simulink model "OFDM_Tx_HW"  (R2020a)
settings: Solver=FixedStepDiscrete  StartTime=0.0  StopTime=inf  RelTol=1e-3
InitFcn:
  | % Set parameters
  | fs = 20e6;
  | fclk = 240e6;
  | ssr = 2;
  | fdc = fclk*ssr*8;
  | 
  | % Load libraries
  | addpath('./lib');
  | 
  | % Create filters
  | run ./filter_design_20mhz;
  | 
  | % Load all required variables
  | load('variables/read_addr_data');
  | load('variables/read_addr_cp');
  | load('variables/read_addr_pream');
  | load('variables/read_addr_rx');
  | load('variables/pilot');
  | load('variables/sc_index');
  | load('variables/LTSfreq');
  | load('variables/STSfreq');
  | load('variables/LTSread');
  | load('variables/STSread');
  | 
  | run ./scripts/rfgen;
values from neighbouring files (symbols this model uses):
  decimation_unique = dsp.SampleRateConverter('InputSampleRate', fdc/64,     'OutputSampleRate', fs,     'Bandwidth', fs*0.9,     'OutputRateTolerance', 0,     'StopbandAttenuation', 100)    [filter_design_20mhz.m]
  interpolation_single = dsp.SampleRateConverter('InputSampleRate', fs,     'OutputSampleRate', fclk,     'Bandwidth', fs*0.9,     'OutputRateTolerance', 0,     'StopbandAttenuation', 100)    [filter_design_20mhz.m]
  interpolation_ssr = dsp.SampleRateConverter('InputSampleRate', fclk,     'OutputSampleRate', fclk*ssr,     'Bandwidth', fs*0.9,     'OutputRateTolerance', 0,     'StopbandAttenuation', 100)    [filter_design_20mhz.m]
undefined symbols (not defined in the file or in its folder): designMultirateFIR, LTSfreq, LTSread, pilot, read_addr_cp, read_addr_data, read_addr_pream, read_addr_rx, sc_index, STSfreq, STSread
libraries: hdlsllib x87, simulink x55, xbsIndex_r4 x48, dspmlti4 x23, xrbsSSR_Library x8, dspsigops x6, dspswit3 x4, dsphdlmathfun x3, dspsigattribs x2, dsphdlxfrm x2, dsphdlsigops x1, lib_rfsignalgenerator x1
(part 2 of 6)

== system OFDM_Tx_HW/OFDMTx/DataGenerator ==
  modScheme : Inport
  dataValid : Inport  Port=2
  preambleValid : Inport  Port=3
  dataReady : Inport  Port=4
  pilotValid : Inport  Port=5
  Constant : Constant  Value=0  OutDataTypeStr=boolean  SampleTime=1/fs
  Data Multiplexer : MATLAB Function  TreatAsAtomicUnit=on
  LTSfreq : Subsystem
  PilotGen : Subsystem
  RF Signal Generator : lib_rfsignalgenerator/RF Signal Generator  SystemSampleTime=-1  Latency=0  AutoFrameSizeCalculation=off
  STSFreq : Subsystem
  dataOut : Outport  VectorParamsAs1DForOutWhenUnconnected=off
  preambValOut : Outport  Port=2  VectorParamsAs1DForOutWhenUnconnected=off
  dataValidOut : Outport  Port=3  VectorParamsAs1DForOutWhenUnconnected=off
  symValidOut : Outport  Port=4  VectorParamsAs1DForOutWhenUnconnected=off
  wires:
  dataValid/1 -> PilotGen/1(dataValidIn), dataValidOut/1
  preambleValid/1 -> STSFreq/1(preamVal), LTSfreq/1(preambVal), preambValOut/1
  LTSfreq/2(ltsVal) -> Data Multiplexer/8(ltsval)
  LTSfreq/1(ltsFreq) -> Data Multiplexer/7(lts)
  STSFreq/2(stsVal) -> Data Multiplexer/6(stsval)
  STSFreq/1(stsFreq) -> Data Multiplexer/5(sts)
  pilotValid/1 -> PilotGen/2(pilotValidIn), Data Multiplexer/4(pval)
  PilotGen/1(pilotOut) -> Data Multiplexer/3(pilots)
  RF Signal Generator/2 -> Data Multiplexer/1(symbols)
  Data Multiplexer/1(data) -> dataOut/1
  modScheme/1 -> RF Signal Generator/1
  RF Signal Generator/1 -> symValidOut/1
  Constant/1 -> RF Signal Generator/2
  dataReady/1 -> RF Signal Generator/3, Data Multiplexer/2(dataready)

== system OFDM_Tx_HW/OFDMTx/IFFT ==
  dataIn : Inport
  preambleValidIn : Inport  Port=2
  "dataValidIn " : Inport  Port=3
  Delay : Delay  DelayLength=173  InitialCondition=0  UseCircularBuffer=on
  Delay1 : Delay  DelayLength=173  InitialCondition=0  UseCircularBuffer=on
  IFFT HDL Optimized : dsphdlxfrm/IFFT HDL Optimized  FFTLength=64  Architecture=Streaming Radix 2^2  ComplexMultiplication=Use 3 multipliers and 5 adders  BitReversedOutput=off  BitReversedInput=off  Normalize=on  SimulateUsing=Code generation  RoundingMethod=Floor  ResetInputPort=off  StartOutputPort=off  EndOutputPort=off
      settings: SourceProductBaseCode=DS
  IFFTValid : Subsystem
  Terminator : Terminator
  dataOut : Outport  VectorParamsAs1DForOutWhenUnconnected=off
  preambValidOut : Outport  Port=2  VectorParamsAs1DForOutWhenUnconnected=off
  dataValidOut : Outport  Port=3  VectorParamsAs1DForOutWhenUnconnected=off
  wires:
  dataIn/1 -> IFFT HDL Optimized/1
  IFFT HDL Optimized/2 -> Terminator/1
  "dataValidIn "/1 -> IFFTValid/2(dataValid), Delay1/1
  IFFTValid/1(ifftValid) -> IFFT HDL Optimized/2
  preambleValidIn/1 -> IFFTValid/1(preambleValid), Delay/1
  Delay/1 -> preambValidOut/1
  Delay1/1 -> dataValidOut/1
  IFFT HDL Optimized/1 -> dataOut/1

== system OFDM_Tx_HW/OFDMTx/SCMapper ==
  dataIn : Inport
  preambValid : Inport  Port=2
  dataValid : Inport  Port=3
  DataMapper : Subsystem
  Mux2 : MATLAB Function  TreatAsAtomicUnit=on
  PremableMapper : Subsystem
  dataOut : Outport  VectorParamsAs1DForOutWhenUnconnected=off
  preambValidOut : Outport  Port=2  VectorParamsAs1DForOutWhenUnconnected=off
  dataValidOut : Outport  Port=3  VectorParamsAs1DForOutWhenUnconnected=off
  wires:
  PremableMapper/1(preambleShiftOut) -> Mux2/1(preamb)
  PremableMapper/2(preambValOut) -> preambValidOut/1, Mux2/2(preambVal)
  DataMapper/1(dataOut) -> Mux2/3(data)
  DataMapper/2(dataValidOut) -> dataValidOut/1, Mux2/4(dataVal)
  dataIn/1 -> DataMapper/1(dataIn), PremableMapper/1(data)
  preambValid/1 -> PremableMapper/2(preambVal)
  dataValid/1 -> DataMapper/2(dataValid)
  Mux2/1(dataOut) -> dataOut/1

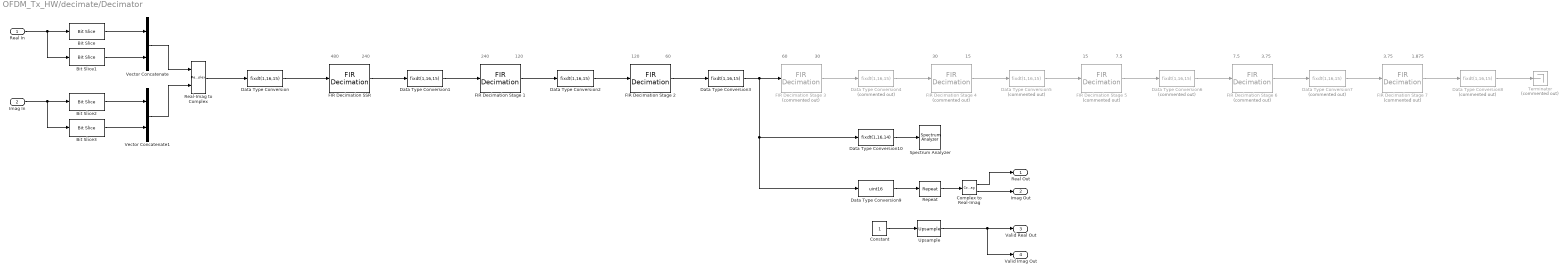
== system OFDM_Tx_HW/decimate/Decimator ==
  note: 1.875
  note: 3.75
  note: 3.75
  note: 7.5
  note: 7.5
  note: 15
  note: 15
  note: 30
  note: 30
  note: 480
  note: 240
  note: 240
  note: 120
  note: 120
  note: 60
  note: 60
  Real In : Inport
  Imag In : Inport  Port=2
  Bit Slice : hdlsllib/Logic and Bit Operations/Bit Slice  lidx=15  ridx=0
      settings: SourceProductBaseCode=SL
  Bit Slice1 : hdlsllib/Logic and Bit Operations/Bit Slice  lidx=31  ridx=16
      settings: SourceProductBaseCode=SL
  Bit Slice2 : hdlsllib/Logic and Bit Operations/Bit Slice  lidx=15  ridx=0
      settings: SourceProductBaseCode=SL
  Bit Slice3 : hdlsllib/Logic and Bit Operations/Bit Slice  lidx=31  ridx=16
      settings: SourceProductBaseCode=SL
  Complex to Real-Imag : ComplexToRealImag
  Constant : Constant  OutDataTypeStr=boolean  SampleTime=1/(fclk/4)
  Data Type Conversion : DataTypeConversion  OutDataTypeStr=fixdt(1,16,15)  ConvertRealWorld=Stored Integer (SI)
  Data Type Conversion1 : DataTypeConversion  OutDataTypeStr=fixdt(1,16,15)  RndMeth=Round  SaturateOnIntegerOverflow=on
  Data Type Conversion10 : DataTypeConversion  OutDataTypeStr=fixdt(1,16,14)  ConvertRealWorld=Stored Integer (SI)
  Data Type Conversion2 : DataTypeConversion  OutDataTypeStr=fixdt(1,16,15)  RndMeth=Round  SaturateOnIntegerOverflow=on
  Data Type Conversion3 : DataTypeConversion  OutDataTypeStr=fixdt(1,16,15)  RndMeth=Round  SaturateOnIntegerOverflow=on
  Data Type Conversion{4..8} (5 alike) : DataTypeConversion  Commented=on  OutDataTypeStr=fixdt(1,16,15)  RndMeth=Round  SaturateOnIntegerOverflow=on
  Data Type Conversion9 : DataTypeConversion  OutDataTypeStr=uint16  ConvertRealWorld=Stored Integer (SI)
  FIR Decimation SSR : dspmlti4/FIR Decimation  FilterSource=Dialog parameters  h=decimation_ssr.Numerator  D=2  filtStruct=Direct form  FilterObject=FDECIM  InputProcessing=Columns as channels (frame based)  framing=Enforce single-rate processing  inputOffset=0  outputBufInitCond=0  roundingMode=Floor  overflowMode=off  firstCoeffDataTypeStr=Inherit: Same word length as input  firstCoeffMin=[]  firstCoeffMax=[]  firstCoeffLastDataTypeStr=Inherit: Same word length as input  outputDataTypeStr=Inherit: Same as product output  outputMin=[]  outputMax=[]  outputLastDataTypeStr=Inherit: Same as product output
  FIR Decimation Stage 1 : dspmlti4/FIR Decimation  FilterSource=Dialog parameters  h=decimation_single.Numerator  D=2  filtStruct=Direct form  FilterObject=FDECIM  framing=Enforce single-rate processing  inputOffset=0  outputBufInitCond=0  roundingMode=Floor  overflowMode=off  firstCoeffDataTypeStr=Inherit: Same word length as input  firstCoeffMin=[]  firstCoeffMax=[]  firstCoeffLastDataTypeStr=Inherit: Same word length as input  outputDataTypeStr=Inherit: Same as product output  outputMin=[]  outputMax=[]  outputLastDataTypeStr=Inherit: Same as product output
  FIR Decimation Stage 2 : dspmlti4/FIR Decimation  FilterSource=Dialog parameters  h=decimation_single.Numerator  D=2  filtStruct=Direct form  FilterObject=FDECIM  framing=Enforce single-rate processing  inputOffset=0  outputBufInitCond=0  roundingMode=Floor  overflowMode=off  firstCoeffDataTypeStr=Inherit: Same word length as input  firstCoeffMin=[]  firstCoeffMax=[]  firstCoeffLastDataTypeStr=Inherit: Same word length as input  outputDataTypeStr=Inherit: Same as product output  outputMin=[]  outputMax=[]  outputLastDataTypeStr=Inherit: Same as product output
  FIR Decimation Stage {3..7} (5 alike) : dspmlti4/FIR Decimation  Commented=on  FilterSource=Dialog parameters  h=decimation_single.Numerator  D=2  filtStruct=Direct form  FilterObject=FDECIM  framing=Enforce single-rate processing  inputOffset=0  outputBufInitCond=0  roundingMode=Floor  overflowMode=off  firstCoeffDataTypeStr=Inherit: Same word length as input  firstCoeffMin=[]  firstCoeffMax=[]  firstCoeffLastDataTypeStr=Inherit: Same word length as input  outputDataTypeStr=Inherit: Same as product output  outputMin=[]  outputMax=[]  outputLastDataTypeStr=Inherit: Same as product output
  Real-Imag to Complex : RealImagToComplex
  Repeat : dspsigops/Repeat  N=4  RateOptions=Allow multirate processing  ic=0  mode=Unused parameter value
  Spectrum Analyzer : SpectrumAnalyzer
  Terminator : Terminator  Commented=on
  Upsample : dspsigops/Upsample  N=4  phase=0  RateOptions=Allow multirate processing  ic=0  mode=Unused parameter value
  Vector Concatenate : Concatenate
  Vector Concatenate1 : Concatenate
  Real Out : Outport
  Imag Out : Outport  Port=2
  Valid Real Out : Outport  Port=3
  Valid Imag Out : Outport  Port=4
  wires:
  Data Type Conversion8/1 -> Terminator/1
  Data Type Conversion3/1 -> Data Type Conversion10/1, Data Type Conversion9/1, FIR Decimation Stage 3/1
  Data Type Conversion10/1 -> Spectrum Analyzer/1
  Upsample/1 -> Valid Real Out/1, Valid Imag Out/1
  Data Type Conversion9/1 -> Repeat/1
  Repeat/1 -> Complex to Real-Imag/1
  Data Type Conversion2/1 -> FIR Decimation Stage 2/1
  FIR Decimation Stage 6/1 -> Data Type Conversion7/1
  Data Type Conversion1/1 -> FIR Decimation Stage 1/1
  FIR Decimation Stage 1/1 -> Data Type Conversion2/1
  Complex to Real-Imag/2 -> Imag Out/1
  Vector Concatenate1/1 -> Real-Imag to Complex/2
  Vector Concatenate/1 -> Real-Imag to Complex/1
  Real-Imag to Complex/1 -> Data Type Conversion/1
  Bit Slice1/1 -> Vector Concatenate/2
  FIR Decimation Stage 5/1 -> Data Type Conversion6/1
  Bit Slice/1 -> Vector Concatenate/1
  FIR Decimation SSR/1 -> Data Type Conversion1/1
  FIR Decimation Stage 7/1 -> Data Type Conversion8/1
  Real In/1 -> Bit Slice/1, Bit Slice1/1
  Data Type Conversion6/1 -> FIR Decimation Stage 6/1
  FIR Decimation Stage 2/1 -> Data Type Conversion3/1
  Data Type Conversion7/1 -> FIR Decimation Stage 7/1
  Bit Slice2/1 -> Vector Concatenate1/1
  Constant/1 -> Upsample/1
  Imag In/1 -> Bit Slice3/1, Bit Slice2/1
  FIR Decimation Stage 4/1 -> Data Type Conversion5/1
  Data Type Conversion/1 -> FIR Decimation SSR/1
  Bit Slice3/1 -> Vector Concatenate1/2
  FIR Decimation Stage 3/1 -> Data Type Conversion4/1
  Complex to Real-Imag/1 -> Real Out/1
  Data Type Conversion5/1 -> FIR Decimation Stage 5/1
  Data Type Conversion4/1 -> FIR Decimation Stage 4/1

== system OFDM_Tx_HW/decimate/Unique Decimation ==
  Real In : Inport
  Imag In : Inport  Port=2
  Valid Real In : Inport  Port=3
  Valid Imag In : Inport  Port=4
  Unique Decimation : Subsystem  VariantControl=SystemGenerator
  Unique Decimation1 : Subsystem  VariantControl=Simulink
  Data : Outport
  Valid : Outport  Port=2

== system OFDM_Tx_HW/interpolate/interpolate ==
  s_tdata : Inport
  s_tvalid : Inport  Port=2
  Convert To AXI-Stream : Subsystem
  Data Type Conversion2 : DataTypeConversion  OutDataTypeStr=uint64
  Data Type Conversion8 : DataTypeConversion  OutDataTypeStr=boolean
  FIR Interpolation SSR : Subsystem
  FIR Interpolation Single : Subsystem
  Imag Slice : xbsIndex_r4/Slice  nbits=1  boolean_output=off  mode=Two Bit Locations  bit1=31  base1=LSB of Input  bit0=16  base0=LSB of Input  dbl_ovrd=off  block_type=slice
  Real Slice : xbsIndex_r4/Slice  nbits=1  boolean_output=off  mode=Two Bit Locations  bit1=15  base1=LSB of Input  bit0=0  base0=LSB of Input  dbl_ovrd=off  block_type=slice
  Reinterpret : xbsIndex_r4/Reinterpret  force_arith_type=on  arith_type="Signed  (2's comp)"  force_bin_pt=on  bin_pt=14  block_type=reinterpret
  Reinterpret1 : xbsIndex_r4/Reinterpret  force_arith_type=on  arith_type="Signed  (2's comp)"  force_bin_pt=on  bin_pt=14  block_type=reinterpret
  Terminator : Terminator
  data : xbsIndex_r4/Gateway In  gui_display_data_type=Fixed-point  arith_type=Unsigned  n_bits=32  bin_pt=0  preci_type=Single  exp_width=8  frac_width=24  rows=1  columns=1  quantization="Round  (unbiased: +/- Inf)"  overflow=Saturate  period=1/(fs)  UseAsADC=off  ADCChannel='1'  interface=None  automatic_assignment=on  address_offset=hex2dec('00')  intf_name=''  intf_description=''  default_value=0  timing_constraint=None  locs_specified=off  LOCs={}  io_standard={}  inherit_from_input=off  hdl_port=on  dbl_ovrd=off  block_type=gatewayin
  m_axis_tdata : xbsIndex_r4/Gateway Out  inherit_from_input=on  hdl_port=on  rows=1  columns=1  UseAsDAC=off  DACChannel='1'  interface=None  automatic_assignment=on  address_offset=hex2dec('00')  intf_name=''  intf_description=''  timing_constraint=None  locs_specified=off  LOCs={}  io_standard={}  block_type=gatewayout
  m_axis_tvalid : xbsIndex_r4/Gateway Out  inherit_from_input=off  hdl_port=on  rows=1  columns=1  UseAsDAC=off  DACChannel='1'  interface=None  automatic_assignment=on  address_offset=hex2dec('00')  intf_name=''  intf_description=''  timing_constraint=None  locs_specified=off  LOCs={}  io_standard={}  block_type=gatewayout
  valid : xbsIndex_r4/Gateway In  gui_display_data_type=Boolean  arith_type=Boolean  n_bits=32  bin_pt=0  preci_type=Single  exp_width=8  frac_width=24  rows=1  columns=1  quantization="Round  (unbiased: +/- Inf)"  overflow=Saturate  period=1/(fs)  UseAsADC=off  ADCChannel='1'  interface=None  automatic_assignment=on  address_offset=hex2dec('00')  intf_name=''  intf_description=''  default_value=0  timing_constraint=None  locs_specified=off  LOCs={}  io_standard={}  inherit_from_input=off  hdl_port=on  dbl_ovrd=off  block_type=gatewayin
  m_tdata : Outport
  m_tvalid : Outport  Port=2
  wires:
  Data Type Conversion8/1 -> m_tvalid/1
  s_tvalid/1 -> valid/1
  Data Type Conversion2/1 -> m_tdata/1
  m_axis_tdata/1 -> Data Type Conversion2/1
  m_axis_tvalid/1 -> Data Type Conversion8/1
  s_tdata/1 -> data/1
  valid/1 -> Terminator/1
  data/1 -> Imag Slice/1, Real Slice/1
  Real Slice/1 -> Reinterpret/1
  Imag Slice/1 -> Reinterpret1/1
  Reinterpret/1 -> FIR Interpolation Single/1(Real In)
  Reinterpret1/1 -> FIR Interpolation Single/2(Imag In)
  FIR Interpolation Single/1(Real Out) -> FIR Interpolation SSR/1(Real In)
  FIR Interpolation Single/2(Imag Out) -> FIR Interpolation SSR/2(Imag In)
  FIR Interpolation SSR/1(Real Out) -> Convert To AXI-Stream/1(Real In)
  FIR Interpolation SSR/2(Imag Out) -> Convert To AXI-Stream/2(Imag In)
  Convert To AXI-Stream/1(Data Out) -> m_axis_tdata/1
  Convert To AXI-Stream/2(Valid Out) -> m_axis_tvalid/1

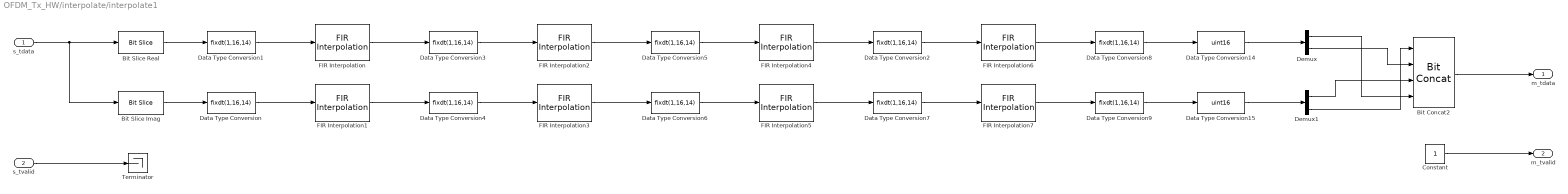
== system OFDM_Tx_HW/interpolate/interpolate1 ==
  s_tdata : Inport
  s_tvalid : Inport  Port=2
  Bit Concat2 : hdlsllib/Logic and Bit Operations/Bit Concat  numInputs=4
  Bit Slice Imag : hdlsllib/Logic and Bit Operations/Bit Slice  lidx=31  ridx=16
      settings: SourceProductBaseCode=SL
  Bit Slice Real : hdlsllib/Logic and Bit Operations/Bit Slice  lidx=15  ridx=0
      settings: SourceProductBaseCode=SL
  Constant : Constant  OutDataTypeStr=boolean  SampleTime=1/fclk
  Data Type Conversion : DataTypeConversion  OutDataTypeStr=fixdt(1,16,14)  ConvertRealWorld=Stored Integer (SI)
  Data Type Conversion1 : DataTypeConversion  OutDataTypeStr=fixdt(1,16,14)  ConvertRealWorld=Stored Integer (SI)
  Data Type Conversion14 : DataTypeConversion  OutDataTypeStr=uint16  ConvertRealWorld=Stored Integer (SI)
  Data Type Conversion15 : DataTypeConversion  OutDataTypeStr=uint16  ConvertRealWorld=Stored Integer (SI)
  Data Type Conversion{2..9} (8 alike) : DataTypeConversion  OutDataTypeStr=fixdt(1,16,14)  RndMeth=Round  SaturateOnIntegerOverflow=on
  Demux : Demux  Outputs=2
  Demux1 : Demux  Outputs=2
  FIR Interpolation : dspmlti4/FIR Interpolation  FilterSource=Dialog parameters  PrivateCoeffs=0  h=interpolation_single.getFilters.Stage1.Numerator  L=interpolation_single.getFilters.Stage1.InterpolationFactor  FilterObject=FINTERP  framing=Allow multirate processing  outputBufInitCond=0  roundingMode=Floor  overflowMode=off  firstCoeffDataTypeStr=Inherit: Same word length as input  firstCoeffMin=[]  firstCoeffMax=[]  firstCoeffLastDataTypeStr=Inherit: Same word length as input  outputDataTypeStr=Inherit: Same as product output  outputMin=[]  outputMax=[]  outputLastDataTypeStr=Inherit: Same as product output
  FIR Interpolation1 : dspmlti4/FIR Interpolation  FilterSource=Dialog parameters  PrivateCoeffs=0  h=interpolation_single.getFilters.Stage1.Numerator  L=interpolation_single.getFilters.Stage1.InterpolationFactor  FilterObject=FINTERP  framing=Allow multirate processing  outputBufInitCond=0  roundingMode=Floor  overflowMode=off  firstCoeffDataTypeStr=Inherit: Same word length as input  firstCoeffMin=[]  firstCoeffMax=[]  firstCoeffLastDataTypeStr=Inherit: Same word length as input  outputDataTypeStr=Inherit: Same as product output  outputMin=[]  outputMax=[]  outputLastDataTypeStr=Inherit: Same as product output
  FIR Interpolation2 : dspmlti4/FIR Interpolation  FilterSource=Dialog parameters  PrivateCoeffs=0  h=interpolation_single.getFilters.Stage2.Numerator  L=interpolation_single.getFilters.Stage2.InterpolationFactor  FilterObject=FINTERP  framing=Enforce single-rate processing  outputBufInitCond=0  roundingMode=Floor  overflowMode=off  firstCoeffDataTypeStr=Inherit: Same word length as input  firstCoeffMin=[]  firstCoeffMax=[]  firstCoeffLastDataTypeStr=Inherit: Same word length as input  outputDataTypeStr=Inherit: Same as product output  outputMin=[]  outputMax=[]  outputLastDataTypeStr=Inherit: Same as product output
  FIR Interpolation3 : dspmlti4/FIR Interpolation  FilterSource=Dialog parameters  PrivateCoeffs=0  h=interpolation_single.getFilters.Stage2.Numerator  L=interpolation_single.getFilters.Stage2.InterpolationFactor  FilterObject=FINTERP  framing=Enforce single-rate processing  outputBufInitCond=0  roundingMode=Floor  overflowMode=off  firstCoeffDataTypeStr=Inherit: Same word length as input  firstCoeffMin=[]  firstCoeffMax=[]  firstCoeffLastDataTypeStr=Inherit: Same word length as input  outputDataTypeStr=Inherit: Same as product output  outputMin=[]  outputMax=[]  outputLastDataTypeStr=Inherit: Same as product output
  FIR Interpolation4 : dspmlti4/FIR Interpolation  FilterSource=Dialog parameters  PrivateCoeffs=0  h=interpolation_single.getFilters.Stage3.Numerator  L=interpolation_single.getFilters.Stage3.InterpolationFactor  FilterObject=FINTERP  framing=Enforce single-rate processing  outputBufInitCond=0  roundingMode=Floor  overflowMode=off  firstCoeffDataTypeStr=Inherit: Same word length as input  firstCoeffMin=[]  firstCoeffMax=[]  firstCoeffLastDataTypeStr=Inherit: Same word length as input  outputDataTypeStr=Inherit: Same as product output  outputMin=[]  outputMax=[]  outputLastDataTypeStr=Inherit: Same as product output
  FIR Interpolation5 : dspmlti4/FIR Interpolation  FilterSource=Dialog parameters  PrivateCoeffs=0  h=interpolation_single.getFilters.Stage3.Numerator  L=interpolation_single.getFilters.Stage3.InterpolationFactor  FilterObject=FINTERP  framing=Enforce single-rate processing  outputBufInitCond=0  roundingMode=Floor  overflowMode=off  firstCoeffDataTypeStr=Inherit: Same word length as input  firstCoeffMin=[]  firstCoeffMax=[]  firstCoeffLastDataTypeStr=Inherit: Same word length as input  outputDataTypeStr=Inherit: Same as product output  outputMin=[]  outputMax=[]  outputLastDataTypeStr=Inherit: Same as product output
  FIR Interpolation6 : dspmlti4/FIR Interpolation  FilterSource=Dialog parameters  PrivateCoeffs=0  h=interpolation_ssr.getFilters.Stage1.Numerator  L=interpolation_ssr.getFilters.Stage1.InterpolationFactor  FilterObject=FINTERP  InputProcessing=Columns as channels (frame based)  framing=Enforce single-rate processing  outputBufInitCond=0  roundingMode=Floor  overflowMode=off  firstCoeffDataTypeStr=Inherit: Same word length as input  firstCoeffMin=[]  firstCoeffMax=[]  firstCoeffLastDataTypeStr=Inherit: Same word length as input  outputDataTypeStr=Inherit: Same as product output  outputMin=[]  outputMax=[]  outputLastDataTypeStr=Inherit: Same as product output
  FIR Interpolation7 : dspmlti4/FIR Interpolation  FilterSource=Dialog parameters  PrivateCoeffs=0  h=interpolation_ssr.getFilters.Stage1.Numerator  L=interpolation_ssr.getFilters.Stage1.InterpolationFactor  FilterObject=FINTERP  InputProcessing=Columns as channels (frame based)  framing=Enforce single-rate processing  outputBufInitCond=0  roundingMode=Floor  overflowMode=off  firstCoeffDataTypeStr=Inherit: Same word length as input  firstCoeffMin=[]  firstCoeffMax=[]  firstCoeffLastDataTypeStr=Inherit: Same word length as input  outputDataTypeStr=Inherit: Same as product output  outputMin=[]  outputMax=[]  outputLastDataTypeStr=Inherit: Same as product output
  Terminator : Terminator
  m_tdata : Outport
  m_tvalid : Outport  Port=2
  wires:
  Data Type Conversion9/1 -> Data Type Conversion15/1
  Data Type Conversion8/1 -> Data Type Conversion14/1
  Data Type Conversion2/1 -> FIR Interpolation6/1
  Data Type Conversion7/1 -> FIR Interpolation7/1
  FIR Interpolation7/1 -> Data Type Conversion9/1
  FIR Interpolation6/1 -> Data Type Conversion8/1
  Data Type Conversion6/1 -> FIR Interpolation5/1
  Data Type Conversion5/1 -> FIR Interpolation4/1
  FIR Interpolation4/1 -> Data Type Conversion2/1
  FIR Interpolation5/1 -> Data Type Conversion7/1
  Demux1/2 -> Bit Concat2/1
  FIR Interpolation/1 -> Data Type Conversion3/1
  Demux/2 -> Bit Concat2/2
  Demux/1 -> Bit Concat2/4
  Data Type Conversion14/1 -> Demux/1
  Data Type Conversion15/1 -> Demux1/1
  FIR Interpolation3/1 -> Data Type Conversion6/1
  Data Type Conversion3/1 -> FIR Interpolation2/1
  FIR Interpolation1/1 -> Data Type Conversion4/1
  Bit Slice Imag/1 -> Data Type Conversion/1
  Data Type Conversion1/1 -> FIR Interpolation/1
  FIR Interpolation2/1 -> Data Type Conversion5/1
  Bit Slice Real/1 -> Data Type Conversion1/1
  s_tdata/1 -> Bit Slice Imag/1, Bit Slice Real/1
  Data Type Conversion4/1 -> FIR Interpolation3/1
  s_tvalid/1 -> Terminator/1
  Data Type Conversion/1 -> FIR Interpolation1/1
  Demux1/1 -> Bit Concat2/3
  Bit Concat2/1 -> m_tdata/1
  Constant/1 -> m_tvalid/1

== system OFDM_Tx_HW/Channel/RF-ADC/Decimation Filter ==
  Data In : Inport
  FIR 0 : dspmlti4/FIR Decimation  FilterSource=Filter object  h=designMultirateFIR(1,2)  D=2  filtStruct=Direct form  FilterObject=fir0  InputProcessing=Columns as channels (frame based)  framing=Allow multirate processing  inputOffset=0  outputBufInitCond=0  roundingMode=Floor  overflowMode=off  firstCoeffDataTypeStr=Inherit: Same word length as input  firstCoeffMin=[]  firstCoeffMax=[]  firstCoeffLastDataTypeStr=Inherit: Same word length as input  outputDataTypeStr=Inherit: Same as accumulator  outputMin=[]  outputMax=[]  outputLastDataTypeStr=Inherit: Same as accumulator
  FIR 1 : dspmlti4/FIR Decimation  Commented=through  FilterSource=Filter object  h=designMultirateFIR(1,2)  D=2  filtStruct=Direct form  FilterObject=fir1  InputProcessing=Columns as channels (frame based)  framing=Allow multirate processing  inputOffset=0  outputBufInitCond=0  roundingMode=Floor  overflowMode=off  firstCoeffDataTypeStr=Inherit: Same word length as input  firstCoeffMin=[]  firstCoeffMax=[]  firstCoeffLastDataTypeStr=Inherit: Same word length as input  outputDataTypeStr=Inherit: Same as accumulator  outputMin=[]  outputMax=[]  outputLastDataTypeStr=Inherit: Same as accumulator
  FIR 2 : dspmlti4/FIR Decimation  Commented=through  FilterSource=Filter object  h=designMultirateFIR(1,2)  D=2  filtStruct=Direct form  FilterObject=fir2  InputProcessing=Columns as channels (frame based)  framing=Allow multirate processing  inputOffset=0  outputBufInitCond=0  roundingMode=Floor  overflowMode=off  firstCoeffDataTypeStr=Inherit: Same word length as input  firstCoeffMin=[]  firstCoeffMax=[]  firstCoeffLastDataTypeStr=Inherit: Same word length as input  outputDataTypeStr=Inherit: Same as accumulator  outputMin=[]  outputMax=[]  outputLastDataTypeStr=Inherit: Same as accumulator
  Data Out : Outport  VectorParamsAs1DForOutWhenUnconnected=off
  wires:
  FIR 2/1 -> Data Out/1
  Data In/1 -> FIR 0/1
  FIR 0/1 -> FIR 1/1
  FIR 1/1 -> FIR 2/1

== system OFDM_Tx_HW/Channel/RF-ADC/NCO and Mixer ==
  Data In : Inport
  Constant1 : Constant  Value=m  OutDataTypeStr=fixdt(0,2,0)  SampleTime=-1
  Data Type Conversion : DataTypeConversion  OutDataTypeStr=fixdt(1,16,15)
  Multiport Switch1 : MultiPortSwitch  DataPortOrder=Zero-based contiguous  zeroidx=on
  RF-ADC Coarse Mixer : Subsystem
  RF-ADC Fine Mixer : Subsystem
  Real-Imag to Complex : RealImagToComplex
  Data Out : Outport  VectorParamsAs1DForOutWhenUnconnected=off
  wires:
  Multiport Switch1/1 -> Data Out/1
  RF-ADC Fine Mixer/1(Data Out) -> Multiport Switch1/4
  Real-Imag to Complex/1 -> Data Type Conversion/1
  RF-ADC Coarse Mixer/1(Data Out) -> Multiport Switch1/3
  Data In/1 -> Real-Imag to Complex/1, RF-ADC Coarse Mixer/1(Data In), RF-ADC Fine Mixer/1(Data In), Real-Imag to Complex/2
  Constant1/1 -> Multiport Switch1/1
  Data Type Conversion/1 -> Multiport Switch1/2

== system OFDM_Tx_HW/Channel/RF-ADC/RF-ADC ==
  Data In : Inport
  Buffer : Buffer  N=ssr  OutputFrames=off
  Data Type Conversion : DataTypeConversion  OutDataTypeStr=fixdt(1,12,11)  SaturateOnIntegerOverflow=on
  Rate Transition : RateTransition  OutPortSampleTime=1/fs
  Data Out : Outport  VectorParamsAs1DForOutWhenUnconnected=off
  wires:
  Rate Transition/1 -> Data Type Conversion/1
  Data In/1 -> Rate Transition/1
  Data Type Conversion/1 -> Buffer/1
  Buffer/1 -> Data Out/1

== system OFDM_Tx_HW/Channel/RF-ADC/SSR Converter RF-ADC ==
  Real In : Inport
  Imag In : Inport  Port=2
  Constant : Constant  OutDataTypeStr=boolean  SampleTime=-1
  Convert 2-D to 1-D : dspsigattribs/Convert 2-D to 1-D
      settings: SourceProductBaseCode=DS
  Convert 2-D to 1-D1 : dspsigattribs/Convert 2-D to 1-D
      settings: SourceProductBaseCode=DS
  Vector to SSR Imag : Subsystem  mask{N=8, hN=8}
      mask prompts: N "Samples per clock cycle:"
      mask init:
      | if ~isequal(get_param(gcb, 'N'), get_param(gcb, 'hN'))
      |     % Delete all blocks except input and output ports
      |     delete_block(setxor(setdiff(...
      |         find_system(gcb,'LookUnderMasks','on'),...
      |         {[gcb, '/Vector'], [gcb, '/SSR']}), gcb));
      | 
      |     % Delete all wires
      |     delete_line(find_system(gcb, 'FindAll', 'on', 'LookUnderMasks',...
      |         'on', 'SearchDepth', 3, 'Type', 'line', 'Connected', 'off'));
      | 
      |     % Add the bit concatenation block
      |     add_block('hdlsllib/Logic and Bit Operations/Bit Concat',...
      |         [gcb, '/Bit Concat'],...
      |         'Position', [155 55 205 330]);
      |     set_param([gcb, '/Bit Concat'], 'numInputs', num2str(N));
      | 
      |     % Add wire to output
      |     add_line(gcb, 'Bit Concat/1', 'SSR/1');
      | 
      |     % Add selector blocks and connect wires
      |     for i = 0:N-1
      |         add_block('simulink/Signal Routing/Selector',...
      |             [gcb, '/Selector', num2str(i)],...
      |             'Position', [0 82+i*90 45 128+i*90]);
      |         set_param([gcb, '/Selector', num2str(i)], 'InputPortWidth', num2str(N), 'IndexParamArray', {num2str(N-i)});
      |         add_line(gcb, 'Vector/1', ['Selector', num2str(i), '/1'],...
      |             'autorouting', 'on');
      |         add_line(gcb, ['Selector', num2str(i), '/1'],...
      |             ['Bit Concat/', num2str(i+1)],...
      |             'autorouting', 'on');
      |     end
      |     
      |     % Set the hidden attribute to prevent unnecessary changes in
      |     % architecture while generating HDL Code.
      |     set_param(gcb, 'hN', get_param(gcb, 'N'));
      | end
      mask DialogControl DescGroupVar Prompt: Vector to SSR
      mask DialogControl DescTextVar Prompt: Convert a vector of inputs into SSR format.
  Vector to SSR Real : Subsystem  mask{N=8, hN=8}
      mask prompts: N "Samples per clock cycle:"
      mask init: same as OFDM_Tx_HW/Channel/RF-ADC/SSR Converter RF-ADC/Vector to SSR Imag
      mask DialogControl DescGroupVar Prompt: Vector to SSR
      mask DialogControl DescTextVar Prompt: Convert a vector of inputs into SSR format.
  Valid Real : Outport
  Valid Imag : Outport  Port=2
  Real Out : Outport  Port=3
  Imag Out : Outport  Port=4
  wires:
  Real In/1 -> Convert 2-D to 1-D/1
  Imag In/1 -> Convert 2-D to 1-D1/1
  Convert 2-D to 1-D/1 -> Vector to SSR Real/1(Vector)
  Convert 2-D to 1-D1/1 -> Vector to SSR Imag/1(Vector)
  Vector to SSR Real/1(SSR) -> Real Out/1
  Vector to SSR Imag/1(SSR) -> Imag Out/1
  Constant/1 -> Valid Imag/1, Valid Real/1

== system OFDM_Tx_HW/Channel/RF-DAC/Interpolation Filter ==
  Data In : Inport
  FIR 0 : dspmlti4/FIR Interpolation  Commented=through  FilterSource=Filter object  PrivateCoeffs=0  h=designMultirateFIR(3,1)  L=2  FilterObject=fir0  InputProcessing=Columns as channels (frame based)  framing=Allow multirate processing  outputBufInitCond=0  roundingMode=Floor  overflowMode=off  firstCoeffDataTypeStr=Inherit: Same word length as input  firstCoeffMin=[]  firstCoeffMax=[]  firstCoeffLastDataTypeStr=Inherit: Same word length as input  outputDataTypeStr=Inherit: Same as accumulator  outputMin=[]  outputMax=[]  outputLastDataTypeStr=Inherit: Same as accumulator
  FIR 1 : dspmlti4/FIR Interpolation  FilterSource=Filter object  PrivateCoeffs=0  h=designMultirateFIR(3,1)  L=2  FilterObject=fir1  InputProcessing=Columns as channels (frame based)  framing=Allow multirate processing  outputBufInitCond=0  roundingMode=Floor  overflowMode=off  firstCoeffDataTypeStr=Inherit: Same word length as input  firstCoeffMin=[]  firstCoeffMax=[]  firstCoeffLastDataTypeStr=Inherit: Same word length as input  outputDataTypeStr=Inherit: Same as accumulator  outputMin=[]  outputMax=[]  outputLastDataTypeStr=Inherit: Same as accumulator
  FIR 2 : dspmlti4/FIR Interpolation  FilterSource=Filter object  PrivateCoeffs=0  h=designMultirateFIR(3,1)  L=2  FilterObject=fir2  InputProcessing=Columns as channels (frame based)  framing=Allow multirate processing  outputBufInitCond=0  roundingMode=Floor  overflowMode=off  firstCoeffDataTypeStr=Inherit: Same word length as input  firstCoeffMin=[]  firstCoeffMax=[]  firstCoeffLastDataTypeStr=Inherit: Same word length as input  outputDataTypeStr=Inherit: Same as accumulator  outputMin=[]  outputMax=[]  outputLastDataTypeStr=Inherit: Same as accumulator
  Data Out : Outport  VectorParamsAs1DForOutWhenUnconnected=off
  wires:
  FIR 2/1 -> FIR 1/1
  Data In/1 -> FIR 2/1
  FIR 0/1 -> Data Out/1
  FIR 1/1 -> FIR 0/1

== system OFDM_Tx_HW/Channel/RF-DAC/NCO and Mixer ==
  Data In : Inport
  Complex to Real-Imag : ComplexToRealImag
  Constant1 : Constant  Value=m  OutDataTypeStr=fixdt(0,2,0)  SampleTime=-1
  Multiport Switch1 : MultiPortSwitch  DataPortOrder=Zero-based contiguous  zeroidx=on
  RF-DAC Coarse Mixer : Subsystem
  RF-DAC Fine Mixer : Subsystem
  Terminator : Terminator
  Data Out : Outport  VectorParamsAs1DForOutWhenUnconnected=off
  wires:
  RF-DAC Coarse Mixer/1(Data Out) -> Multiport Switch1/3
  Constant1/1 -> Multiport Switch1/1
  Data In/1 -> Complex to Real-Imag/1, RF-DAC Coarse Mixer/1(Data In), RF-DAC Fine Mixer/1(Data In)
  Multiport Switch1/1 -> Data Out/1
  RF-DAC Fine Mixer/1(Data Out) -> Multiport Switch1/4
  Complex to Real-Imag/1 -> Multiport Switch1/2
  Complex to Real-Imag/2 -> Terminator/1

== system OFDM_Tx_HW/Channel/RF-DAC/RF-DAC ==
  Data In : Inport
  Cast To Double : DataTypeConversion  OutDataTypeStr=double
  Rate Transition : RateTransition  OutPortSampleTime=0
  Unbuffer : Unbuffer
  Data Out : Outport  VectorParamsAs1DForOutWhenUnconnected=off
  wires:
  Cast To Double/1 -> Rate Transition/1
  Unbuffer/1 -> Cast To Double/1
  Data In/1 -> Unbuffer/1
  Rate Transition/1 -> Data Out/1

== system OFDM_Tx_HW/Channel/RF-DAC/SSR Converter RF-DAC ==
  Valid : Inport
  Data : Inport  Port=2
  Bit Slice Imag1 : hdlsllib/Logic and Bit Operations/Bit Slice  lidx=31  ridx=16
      settings: SourceProductBaseCode=SL
  Bit Slice Real1 : hdlsllib/Logic and Bit Operations/Bit Slice  lidx=15  ridx=0
      settings: SourceProductBaseCode=SL
  Data Type Conversion : DataTypeConversion  OutDataTypeStr=fixdt(1,16,15)  ConvertRealWorld=Stored Integer (SI)
  Real-Imag to Complex1 : RealImagToComplex
  SSR to Vector Low : Subsystem  mask{N=ssr, w=32, hN=ssr, hw=32}
      mask prompts: N "Samples per clock cycle:"; w "Wordlength:"
      mask init:
      | if ~isequal(get_param(gcb, 'N'), get_param(gcb, 'hN')) ||...
      |         ~isequal(get_param(gcb, 'w'), get_param(gcb, 'hw'))
      |     % Delete all blocks except input and output ports
      |     delete_block(setxor(setdiff(...
      |         find_system(gcb,'LookUnderMasks','on'),...
      |         {[gcb, '/Vector'], [gcb, '/SSR']}), gcb));
      | 
      |     % Delete all wires
      |     delete_line(find_system(gcb, 'FindAll', 'on', 'LookUnderMasks',...
      |         'on', 'SearchDepth', 3, 'Type', 'line', 'Connected', 'off'));
      | 
      |     % Add the matrix concatenation block
      |     add_block('hdlsllib/Math Operations/Matrix Concatenate',...
      |         [gcb, '/Matrix Concatenate'],...
      |         'Position', [155 55 205 330]);
      |     set_param([gcb, '/Matrix Concatenate'], 'NumInputs', num2str(N));
      |     set_param([gcb, '/Matrix Concatenate'], 'ConcatenateDimension', num2str(1));
      |     
      |     % Add wire to output
      |     add_line(gcb, 'Matrix Concatenate/1', 'Vector/1');
      | 
      |     % Add slice blocks and connect wires
      |     for i = 0:N-1
      |         add_block('hdlsllib/Logic and Bit Operations/Bit Slice',...
      |             [gcb, '/Bit Slice', num2str(i)],...
      |             'Position', [0 82+i*90 45 128+i*90]);
      |         set_param([gcb, '/Bit Slice', num2str(i)], 'ridx', num2str(0+i*(w)));
      |         set_param([gcb, '/Bit Slice', num2str(i)], 'lidx', num2str((w-1)+i*(w)));
      |         add_line(gcb, 'SSR/1', ['Bit Slice', num2str(i), '/1'],...
      |             'autorouting', 'on');
      |         add_line(gcb, ['Bit Slice', num2str(i), '/1'],...
      |             ['Matrix Concatenate/', num2str(i+1)],...
      |             'autorouting', 'on');
      |     end
      |     
      |     % Set the hidden attribute to prevent unnecessary changes in
      |     % architecture while generating HDL Code.
      |     set_param(gcb, 'hN', get_param(gcb, 'N'));
      |     set_param(gcb, 'hw', get_param(gcb, 'w'));
      | end
      mask DialogControl DescGroupVar Prompt: SSR to Vector
      mask DialogControl DescTextVar Prompt: Convert the SSR vector format based on the wordlength and expected number of samples per clock cycle.
  Terminator : Terminator
  Data Out : Outport
  wires:
  Data/1 -> SSR to Vector Low/1(SSR)
  Bit Slice Imag1/1 -> Real-Imag to Complex1/2
  Bit Slice Real1/1 -> Real-Imag to Complex1/1
  SSR to Vector Low/1(Vector) -> Bit Slice Imag1/1, Bit Slice Real1/1
  Data Type Conversion/1 -> Data Out/1
  Valid/1 -> Terminator/1
  Real-Imag to Complex1/1 -> Data Type Conversion/1

== system OFDM_Tx_HW/OFDMRx/ChannelEstEq/ChannelEstimate ==
  note: Get and store the channel estimate using the two
      | repetitions of the L-LTF
  note: Write averaged channel estimate to RAM and read out when data is valid
      | for equalisation of successive OFDM symbols.
  note: Note the preamble symbols do not pass this point.
  dataIn : Inport
  preambleValid : Inport  Port=2
  dataValidIn : Inport  Port=3
  ChanEst : Subsystem
  Delay : Delay  DelayLength=5
  Delay1 : Delay  DelayLength=5
  Delay2 : Delay  DelayLength=1
  Dual Port RAM1 : hdlsllib/HDL RAMs/Dual Port RAM  ram_size=6
      settings: SourceProductBaseCode=SL
  HDL Counter3 : hdlsllib/Sources/HDL Counter  CountType=Count limited  CountInit=0  CountStep=1  CountMax=63  CountFromType=Initial value  CountFrom=0  CountResetPort=off  CountLoadPort=off  CountEnbPort=on  CountDirPort=off  CountDataType=Unsigned  CountWordLen=6  CountFracLen=0  CountSampTime=1
  Terminator : Terminator
  WriteEnbAddrGen : Subsystem
  chEstOut : Outport  VectorParamsAs1DForOutWhenUnconnected=off
  dataValidOut : Outport  Port=2  VectorParamsAs1DForOutWhenUnconnected=off
  wires:
  Dual Port RAM1/1 -> Terminator/1
  WriteEnbAddrGen/2(Out2) -> Dual Port RAM1/3
  WriteEnbAddrGen/1(Out1) -> Dual Port RAM1/2
  Delay/1 -> WriteEnbAddrGen/1(In1)
  Delay1/1 -> Delay2/1, HDL Counter3/1
  dataValidIn/1 -> Delay1/1
  ChanEst/1(ChEstOut) -> Dual Port RAM1/1
  dataIn/1 -> ChanEst/1(ChanEstIn)
  preambleValid/1 -> Delay/1, ChanEst/2(PreambValidIn)
  Delay2/1 -> dataValidOut/1
  Dual Port RAM1/2 -> chEstOut/1
  HDL Counter3/1 -> Dual Port RAM1/4

== system OFDM_Tx_HW/OFDMRx/ChannelEstEq/Equalise ==
  note: Perform a complex division to obtain equalised data symbols.
  dataInEq : Inport
  chEstIn : Inport  Port=2
  dataValidIn : Inport  Port=3
  Abs2 : Subsystem
  Complex Mult : Subsystem
  Delay1 : Delay
  Delay8 : Delay  DelayLength=3
  Divide : Subsystem
  dataOutEq : Outport  VectorParamsAs1DForOutWhenUnconnected=off
  dataValidOut : Outport  Port=2  VectorParamsAs1DForOutWhenUnconnected=off
  wires:
  Divide/1(dataOutEq) -> dataOutEq/1
  Delay1/1 -> dataValidOut/1
  Delay8/1 -> Delay1/1
  Abs2/1(Out1) -> Divide/2(In2)
  Complex Mult/1(Out1) -> Divide/1(In1)
  dataInEq/1 -> Complex Mult/1(In1)
  chEstIn/1 -> Complex Mult/2(In2), Abs2/1(ChEstIn)
  dataValidIn/1 -> Delay8/1

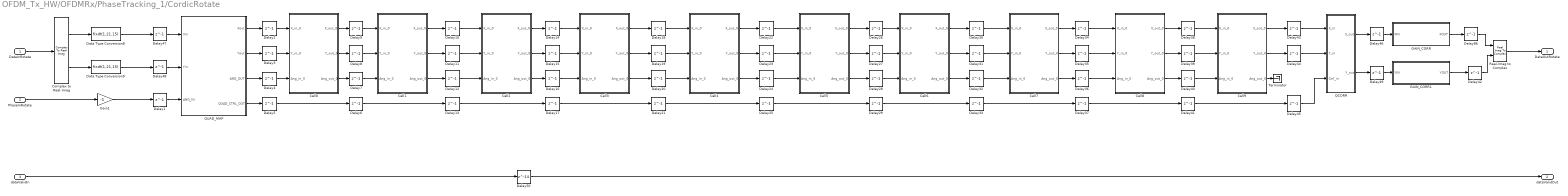
== system OFDM_Tx_HW/OFDMRx/PhaseTracking_1/CordicRotate ==
  DataInRotate : Inport
  PhaseInRotate : Inport  Port=2
  dataValidIn : Inport  Port=3
  Cell0 : Subsystem
  Cell1 : Subsystem
  Cell2 : Subsystem
  Cell3 : Subsystem
  Cell4 : Subsystem
  Cell5 : Subsystem
  Cell6 : Subsystem
  Cell7 : Subsystem
  Cell8 : Subsystem
  Cell9 : Subsystem
  Complex to Real-Imag : ComplexToRealImag
  Data Type Conversion8 : DataTypeConversion  OutDataTypeStr=fixdt(1,21,15)
  Data Type Conversion9 : DataTypeConversion  OutDataTypeStr=fixdt(1,21,15)
  Delay{1..49,86} (50 alike) : Delay  DelayLength=1
  Delay50 : Delay  DelayLength=14
  GAIN_CORR : Subsystem
  GAIN_CORR1 : Subsystem
  Gain1 : Gain  Gain=-1  OutDataTypeStr=fixdt(1,23,20)
  QCORR : Subsystem
  QUAD_MAP : Subsystem
  Real-Imag to Complex : RealImagToComplex
  Terminator : Terminator
  "DataOutRotate  " : Outport  VectorParamsAs1DForOutWhenUnconnected=off
  dataValidOut : Outport  Port=2  VectorParamsAs1DForOutWhenUnconnected=off
  wires:
  Real-Imag to Complex/1 -> "DataOutRotate  "/1
  Delay42/1 -> Real-Imag to Complex/2
  Delay86/1 -> Real-Imag to Complex/1
  Complex to Real-Imag/1 -> Data Type Conversion8/1
  DataInRotate/1 -> Complex to Real-Imag/1
  Complex to Real-Imag/2 -> Data Type Conversion9/1
  GAIN_CORR/1(XOUT) -> Delay86/1
  Delay48/1 -> QUAD_MAP/2(Yin)
  Delay47/1 -> QUAD_MAP/1(Xin)
  QUAD_MAP/1(Xout) -> Delay2/1
  QUAD_MAP/2(Yout) -> Delay3/1
  QUAD_MAP/3(ANG_OUT) -> Delay4/1
  Delay2/1 -> Cell0/1(X_in_0)
  Delay3/1 -> Cell0/2(Y_in_0)
  QUAD_MAP/4(QUAD_CTRL_OUT) -> Delay5/1
  Cell0/1(X_out_0) -> Delay9/1
  Cell0/2(Y_out_0) -> Delay8/1
  Cell0/3(Ang_out_0) -> Delay7/1
  Delay5/1 -> Delay6/1
  Delay7/1 -> Cell1/3(Ang_in_0)
  Delay8/1 -> Cell1/2(Y_in_0)
  Delay9/1 -> Cell1/1(X_in_0)
  Cell1/1(X_out_0) -> Delay10/1
  Cell1/2(Y_out_0) -> Delay11/1
  Cell1/3(Ang_out_0) -> Delay12/1
  Delay6/1 -> Delay13/1
  Delay10/1 -> Cell2/1(X_in_0)
  Delay11/1 -> Cell2/2(Y_in_0)
  Delay12/1 -> Cell2/3(Ang_in_0)
  Delay16/1 -> Cell3/3(Ang_in_0)
  Delay15/1 -> Cell3/2(Y_in_0)
  Delay14/1 -> Cell3/1(X_in_0)
  Delay13/1 -> Delay17/1
  Cell2/3(Ang_out_0) -> Delay16/1
  Cell2/2(Y_out_0) -> Delay15/1
  Cell2/1(X_out_0) -> Delay14/1
  Cell3/1(X_out_0) -> Delay18/1
  Cell3/2(Y_out_0) -> Delay19/1
  Cell3/3(Ang_out_0) -> Delay20/1
  Delay17/1 -> Delay21/1
  Delay18/1 -> Cell4/1(X_in_0)
  Delay19/1 -> Cell4/2(Y_in_0)
  Delay20/1 -> Cell4/3(Ang_in_0)
  Delay24/1 -> Cell5/3(Ang_in_0)
  Delay23/1 -> Cell5/2(Y_in_0)
  Delay22/1 -> Cell5/1(X_in_0)
  Delay21/1 -> Delay25/1
  Cell4/3(Ang_out_0) -> Delay24/1
  Cell4/2(Y_out_0) -> Delay23/1
  Cell4/1(X_out_0) -> Delay22/1
  Cell5/1(X_out_0) -> Delay26/1
  Cell5/2(Y_out_0) -> Delay27/1
  Cell5/3(Ang_out_0) -> Delay28/1
  Delay25/1 -> Delay29/1
  Delay26/1 -> Cell6/1(X_in_0)
  Delay27/1 -> Cell6/2(Y_in_0)
  Delay28/1 -> Cell6/3(Ang_in_0)
  Delay32/1 -> Cell7/3(Ang_in_0)
  Delay31/1 -> Cell7/2(Y_in_0)
  Delay30/1 -> Cell7/1(X_in_0)
  Delay29/1 -> Delay33/1
  Cell6/3(Ang_out_0) -> Delay32/1
  Cell6/2(Y_out_0) -> Delay31/1
  Cell6/1(X_out_0) -> Delay30/1
  Cell7/1(X_out_0) -> Delay34/1
  Cell7/2(Y_out_0) -> Delay35/1
  Cell7/3(Ang_out_0) -> Delay36/1
  Delay33/1 -> Delay37/1
  Delay34/1 -> Cell8/1(X_in_0)
  Delay35/1 -> Cell8/2(Y_in_0)
  Delay36/1 -> Cell8/3(Ang_in_0)
  Delay40/1 -> Cell9/3(Ang_in_0)
  Delay39/1 -> Cell9/2(Y_in_0)
  Delay38/1 -> Cell9/1(X_in_0)
  Delay37/1 -> Delay41/1
  Cell8/3(Ang_out_0) -> Delay40/1
  Cell8/2(Y_out_0) -> Delay39/1
  Cell8/1(X_out_0) -> Delay38/1
  GAIN_CORR1/1(YOUT) -> Delay42/1
  Cell9/3(Ang_out_0) -> Terminator/1
  Delay41/1 -> Delay45/1
  Cell9/1(X_out_0) -> Delay43/1
  Cell9/2(Y_out_0) -> Delay44/1
  Delay43/1 -> QCORR/1(X_in)
  Delay44/1 -> QCORR/2(Y_in)
  Delay46/1 -> GAIN_CORR/1(XIN)
  Delay49/1 -> GAIN_CORR1/1(YIN)
  QCORR/2(Y_out) -> Delay49/1
  Delay1/1 -> QUAD_MAP/3(ANG_IN)
  Delay4/1 -> Cell0/3(Ang_in_0)
  Delay45/1 -> QCORR/3(Ctrl_in)
  Data Type Conversion8/1 -> Delay47/1
  Data Type Conversion9/1 -> Delay48/1
  QCORR/1(X_out) -> Delay46/1
  PhaseInRotate/1 -> Gain1/1
  Gain1/1 -> Delay1/1
  dataValidIn/1 -> Delay50/1
  Delay50/1 -> dataValidOut/1

== system OFDM_Tx_HW/OFDMRx/PhaseTracking_1/DataArrange ==
  note: Re-arrange data symbols
  dataIn : Inport
  dataValidIn : Inport  Port=2
  Delay : Delay  DelayLength=64  InitialCondition=0  UseCircularBuffer=on
  Delay3 : Delay  DelayLength=1  InitialCondition=0  UseCircularBuffer=on
  Dual Port RAM : hdlsllib/HDL RAMs/Dual Port RAM  ram_size=7
      settings: SourceProductBaseCode=SL
  HDL Counter : hdlsllib/Sources/HDL Counter  CountType=Count limited  CountInit=0  CountStep=1  CountMax=127  CountFromType=Initial value  CountFrom=0  CountResetPort=off  CountLoadPort=off  CountEnbPort=on  CountDirPort=off  CountDataType=Unsigned  CountWordLen=7  CountFracLen=0  CountSampTime=1
  HDL Counter1 : hdlsllib/Sources/HDL Counter  CountType=Count limited  CountInit=0  CountStep=1  CountMax=127  CountFromType=Initial value  CountFrom=0  CountResetPort=off  CountLoadPort=off  CountEnbPort=on  CountDirPort=off  CountDataType=Unsigned  CountWordLen=7  CountFracLen=0  CountSampTime=1
  READ_ADDRESS : Lookup_n-D  NumberOfTableDimensions=1  LookupTableObject=''  BreakpointsForDimension1=[0:127]  BreakpointsForDimension1FirstPoint=10  BreakpointsForDimension2FirstPoint=10  BreakpointsForDimension1Spacing=12  BreakpointsForDimension2Spacing=12  IndexSearchMethod=Evenly spaced points  Table=read_addr_rx  TableDataTypeStr=fixdt(0,7,0)  InterpMethod=Flat  DiagnosticForOutOfRangeInput=Error  InternalRulePriority=Speed  OutDataTypeStr=fixdt(0,7,0)  RndMeth=Simplest  InputSameDT=on
  READ_CTRL : Subsystem
  Terminator : Terminator
  dataValidGen : Subsystem
  dataOut : Outport  VectorParamsAs1DForOutWhenUnconnected=off
  dataValidOut : Outport  Port=2  VectorParamsAs1DForOutWhenUnconnected=off
  wires:
  dataValidGen/1(dataValidOut) -> dataValidOut/1
  Delay3/1 -> dataValidGen/1(enb)
  READ_ADDRESS/1 -> READ_CTRL/1(In1)
  READ_CTRL/1(Out1) -> Dual Port RAM/4
  Delay/1 -> READ_CTRL/2(In2), Delay3/1, HDL Counter/1
  HDL Counter1/1 -> Dual Port RAM/2
  dataIn/1 -> Dual Port RAM/1
  Dual Port RAM/2 -> dataOut/1
  HDL Counter/1 -> READ_ADDRESS/1
  dataValidIn/1 -> Dual Port RAM/3, HDL Counter1/1, Delay/1
  Dual Port RAM/1 -> Terminator/1

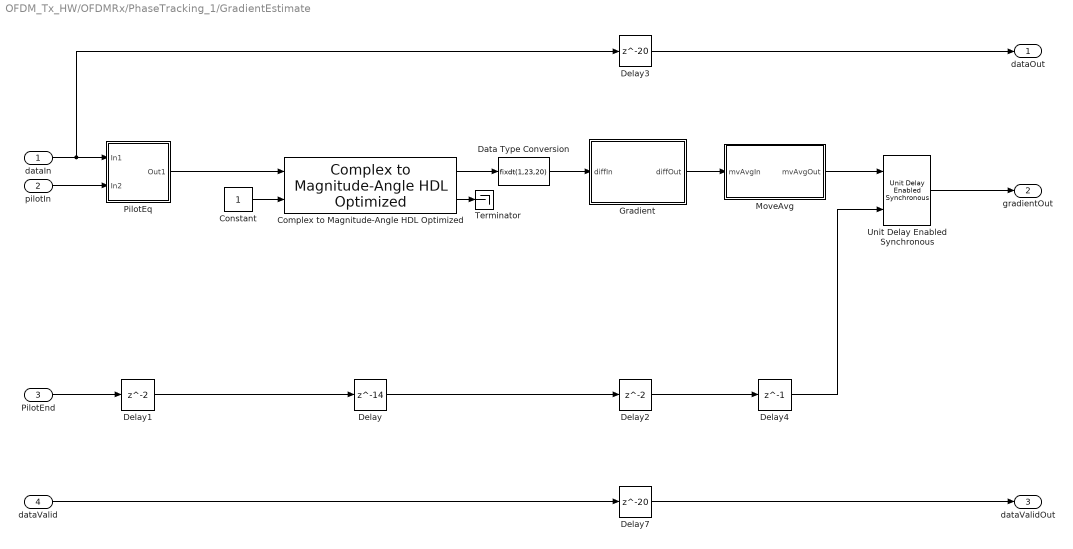
== system OFDM_Tx_HW/OFDMRx/PhaseTracking_1/GradientEstimate  ==
  dataIn : Inport
  pilotIn : Inport  Port=2
  PilotEnd : Inport  Port=3
  dataValid : Inport  Port=4
  Complex to Magnitude-Angle HDL Optimized : dsphdlmathfun/Complex to Magnitude-Angle HDL Optimized  NumIterationsSource=Property  NumIterations=10  OutputFormat=Angle  AngleFormat=Radians  ScaleOutput=off  SimulateUsing=Code generation
      settings: SourceProductBaseCode=DS
  Constant : Constant  OutDataTypeStr=boolean  SampleTime=1/fs
  Data Type Conversion : DataTypeConversion  OutDataTypeStr=fixdt(1,23,20)
  Delay : Delay  DelayLength=14
  Delay1 : Delay
  Delay2 : Delay
  Delay3 : Delay  DelayLength=20
  Delay4 : Delay  DelayLength=1
  Delay7 : Delay  DelayLength=20
  Gradient : Subsystem
  MoveAvg : Subsystem
  PilotEq : Subsystem
  Terminator : Terminator
  Unit Delay Enabled Synchronous : hdlsllib/Discrete/Unit Delay Enabled Synchronous  InitialCondition=0.0  SampleTime=-1
      settings: SourceProductBaseCode=SL
  dataOut : Outport  VectorParamsAs1DForOutWhenUnconnected=off
  gradientOut : Outport  Port=2  VectorParamsAs1DForOutWhenUnconnected=off
  dataValidOut : Outport  Port=3  VectorParamsAs1DForOutWhenUnconnected=off
  wires:
  Delay4/1 -> Unit Delay Enabled Synchronous/2
  Delay/1 -> Delay2/1
  PilotEnd/1 -> Delay1/1
  dataValid/1 -> Delay7/1
  Gradient/1(diffOut) -> MoveAvg/1(mvAvgIn)
  dataIn/1 -> Delay3/1, PilotEq/1(In1)
  pilotIn/1 -> PilotEq/2(In2)
  PilotEq/1(Out1) -> Complex to Magnitude-Angle HDL Optimized/1
  Delay1/1 -> Delay/1
  MoveAvg/1(mvAvgOut) -> Unit Delay Enabled Synchronous/1
  Delay3/1 -> dataOut/1
  Unit Delay Enabled Synchronous/1 -> gradientOut/1
  Delay7/1 -> dataValidOut/1
  Complex to Magnitude-Angle HDL Optimized/1 -> Data Type Conversion/1
  Constant/1 -> Complex to Magnitude-Angle HDL Optimized/2
  Complex to Magnitude-Angle HDL Optimized/2 -> Terminator/1
  Data Type Conversion/1 -> Gradient/1(diffIn)
  Delay2/1 -> Delay4/1

== system OFDM_Tx_HW/OFDMRx/PhaseTracking_1/PhaseErrorEst ==
  dataIn : Inport
  gradientIn : Inport  Port=2
  dataValidIn : Inport  Port=3
  Delay{2..8} (7 alike) : Delay  DelayLength=1
  HDL Counter : hdlsllib/Sources/HDL Counter  CountType=Count limited  CountInit=0  CountStep=1  CountMax=51  CountFromType=Initial value  CountFrom=0  CountResetPort=on  CountLoadPort=off  CountEnbPort=on  CountDirPort=off  CountDataType=Unsigned  CountWordLen=6  CountFracLen=0  CountSampTime=1
  LUT : Lookup_n-D  NumberOfTableDimensions=1  BreakpointsForDimension1=0:51  IndexSearchMethod=Evenly spaced points  Table=sc_index  TableDataTypeStr=fixdt(1,6,0)  InterpMethod=Flat  ExtrapMethod=Clip  DiagnosticForOutOfRangeInput=Error  UseLastTableValue=on  InternalRulePriority=Speed  OutDataTypeStr=fixdt(1,6,0)  RndMeth=Simplest  InputSameDT=on
  NOT : Logic  Operator=NOT  IconShape=distinctive  AllPortsSameDT=off  OutDataTypeStr=boolean
  Product : Product  OutDataTypeStr=fixdt(1,23,20)
  dataOut : Outport  VectorParamsAs1DForOutWhenUnconnected=off
  PhaseOut : Outport  Port=2  VectorParamsAs1DForOutWhenUnconnected=off
  dataValidOut : Outport  Port=3  VectorParamsAs1DForOutWhenUnconnected=off
  wires:
  dataValidIn/1 -> NOT/1, Delay4/1, HDL Counter/2
  dataIn/1 -> Delay2/1
  gradientIn/1 -> Delay3/1
  LUT/1 -> Delay5/1
  NOT/1 -> HDL Counter/1
  HDL Counter/1 -> LUT/1
  Delay3/1 -> Product/1
  Delay5/1 -> Product/2
  Delay2/1 -> Delay6/1
  Delay6/1 -> dataOut/1
  Product/1 -> Delay7/1
  Delay7/1 -> PhaseOut/1
  Delay4/1 -> Delay8/1
  Delay8/1 -> dataValidOut/1

== system OFDM_Tx_HW/OFDMRx/PhaseTracking_1/PilotCtrlGen ==
  dataIn : Inport
  validIn : Inport  Port=2
  CtrlSigGen : Subsystem
  Delay1 : Delay  DelayLength=1
  Delay10 : Delay  DelayLength=1
  SampleCounter : Subsystem
  SymbolCounter : Subsystem
  pilotGen : Subsystem
  dataOut : Outport  VectorParamsAs1DForOutWhenUnconnected=off
  pilotOut : Outport  Port=2  VectorParamsAs1DForOutWhenUnconnected=off
  pilotEnd : Outport  Port=3  VectorParamsAs1DForOutWhenUnconnected=off
  dataValid : Outport  Port=4  VectorParamsAs1DForOutWhenUnconnected=off
  wires:
  Delay1/1 -> pilotGen/3(valid), CtrlSigGen/1(valid)
  SampleCounter/1(Sample_Cnt) -> pilotGen/2(sampleCount), CtrlSigGen/2(sampleCount)
  CtrlSigGen/2(pilotEnd) -> pilotEnd/1
  CtrlSigGen/1(dataValid) -> dataValid/1
  SymbolCounter/1(Symbl_cnt) -> pilotGen/1(symbCount)
  validIn/1 -> Delay1/1, SampleCounter/1(Valid_In), SymbolCounter/1(ValidIn)
  pilotGen/1(pilOut) -> pilotOut/1
  Delay10/1 -> dataOut/1
  dataIn/1 -> Delay10/1
